simulink model "minseg_M2V3_2017a"  (R2017a)
settings: Solver=FixedStepDiscrete  StartTime=0.0  StopTime=inf  FixedStep=mdl_T_sample  RelTol=1e-3
undefined symbols (not defined in the file or in its folder): ctrl_lqr_K2, ctrl_motorDriver_v_ff_cmd_v_val, ctrl_motorDriver_v_ff_cmd_v_val_norm_dx_max, ctrl_motorDriver_v_ff_cmd_v_val_norm_dx_min, ctrl_motorDriver_v_output_max, ctrl_motorDriver_v_output_min, ctrl_motorDriver_v_pid_cmd_thetaDot_val, ctrl_motorDriver_v_pid_cmd_thetaDot_val_norm_dx_max, ctrl_motorDriver_v_pid_cmd_thetaDot_val_norm_dx_min, ctrl_motorDriver_v_pid_int_maxVal, ctrl_motorDriver_v_pid_int_minVal, ctrl_motorDriver_v_pid_k_d, ctrl_motorDriver_v_pid_k_i, ctrl_motorDriver_v_pid_k_p, ctrl_motorDriver_v_rts_ss_k_A, ctrl_motorDriver_v_rts_ss_k_B, ctrl_motorDriver_v_rts_ss_k_C, ctrl_motorDriver_v_rts_ss_k_D, ctrl_motorDriver_v_rts_ss_stateIC, ctrl_motorDriver_v_sfr_cmd_p_x_f, ctrl_motorDriver_v_sfr_cmd_p_x_mag, ctrl_motorDriver_v_sfr_cmd_p_y_f, ctrl_motorDriver_v_sfr_cmd_p_y_mag, ctrl_motorDriver_v_sfr_K, ctrl_motorDriver_v_sfr_K_plant, ctrl_motorDriver_v_sfr_K_rts, ctrl_motorDriver_v_T_cmd, ctrl_motorDriver_v_T_init, DiscIntNeverNeededParam, gyro_bias, io_srl_read_rateTransition_initialCondition, k_intmax_uint8, mdl_T_sample, mtr_encoder_filter_z_ss_A, mtr_encoder_filter_z_ss_B, mtr_encoder_filter_z_ss_C, mtr_encoder_filter_z_ss_D, plant, plant_accel_k_digital2analog, plant_body_l_c, plant_body_l_w, plant_gyro_encoder_filter_z_den, plant_gyro_encoder_filter_z_num, plant_gyro_filter_z_den, plant_gyro_filter_z_num, plant_gyro_k_digital2analog, plant_linear_ss_stateIC, plant_linear_ss_t_A, plant_linear_ss_t_B, plant_linear_ss_t_C, plant_linear_ss_t_D, plant_mtr_encoder_count2wheelRad, plant_mtr_encoder_filter_z_den, plant_mtr_encoder_filter_z_num, plant_pSupply_v, plant_supply_v, plant_T_init, plant_wheel_r
undefined symbols (not defined in the file): ctrl_lqr_addlDyn_A_discrete, ctrl_lqr_addlDyn_B_discrete, ctrl_lqr_addlDyn_C_discrete, ctrl_lqr_addlDyn_D_discrete, ctrl_lqr_addlDyn_k_antiWindup, ctrl_lqr_addlDyn_stateIC, plant_gyro_bias_movingAverage_n_pts, plant_linear_A_continuous, plant_linear_B_continuous, plant_linear_C_continuous, plant_linear_D_continuous, plant_linear_stateIC
libraries: svdutilitieslib x135, simulink x57, arduinolib x15, MinSegLibrary_M2V3 x3, dspindex x3, RASPlib x2
(part 1 of 6)
settings Model: ExtModeTrigDuration=2  Creator=kando  LastModifiedBy=kando
settings DataIOCC: SaveOutput=off  SignalLogging=off  DSMLogging=off  VisualizeSimOutput=off  SaveTime=off
settings OptimizationCC: LifeSpan=Inf  MaxStackSize=64  SimCompilerOptimization=on  AccelVerboseBuild=on
settings DebuggingCC: AllowSymbolicDim=off  SFUnexpectedBacktrackingDiag=warning  SFNoUnconditionalDefaultTransitionDiag=warning  SFExecutionAtInitializationDiag=none
settings HardwareCC: ProdBitPerInt=16  ProdBitPerPointer=16  ProdBitPerSizeT=16  ProdBitPerPtrDiffT=16  ProdLargestAtomicFloat=None  ProdWordSize=8  ProdHWDeviceType=Atmel->AVR  UseEmbeddedCoderFeatures=off  UseSimulinkCoderFeatures=off
settings ModelReferenceCC: PropagateSignalLabelsOutOfModel=off
settings SFSimCC: MATLABDynamicMemAlloc=off
settings RTWCC: SystemTargetFile=ert.tlc  HardwareBoard=Arduino Mega 2560  TLCOptions=-aInlineSetEventsForThisBaseRateFcn=TLC_FALSE -aSuppressMultiTaskScheduler=TLC_FALSE -aRateBasedStepFcn=1  TemplateMakefile=ert_default_tmf  Description=Embedded Coder  Toolchain=Arduino AVR  BuildConfiguration=Faster Runs
settings ERTTargetCC: MultiwordLength=2048  ERTCustomFileBanners=off  SupportContinuousTime=on  SupportNonInlinedSFcns=on  RemoveResetFunc=off  SupportVariableSizeSignals=on  ModelStepFunctionPrototypeControlCompliant=off  ConvertIfToSwitch=off  SuppressUnreachableDefaultCases=off
settings ConfigComp: CovMetricSettings=dw  CovHtmlReporting=on  CovSaveCumulativeToWorkspaceVar=on  CovSaveSingleToWorkspaceVar=on  CovExternalEMLEnable=off

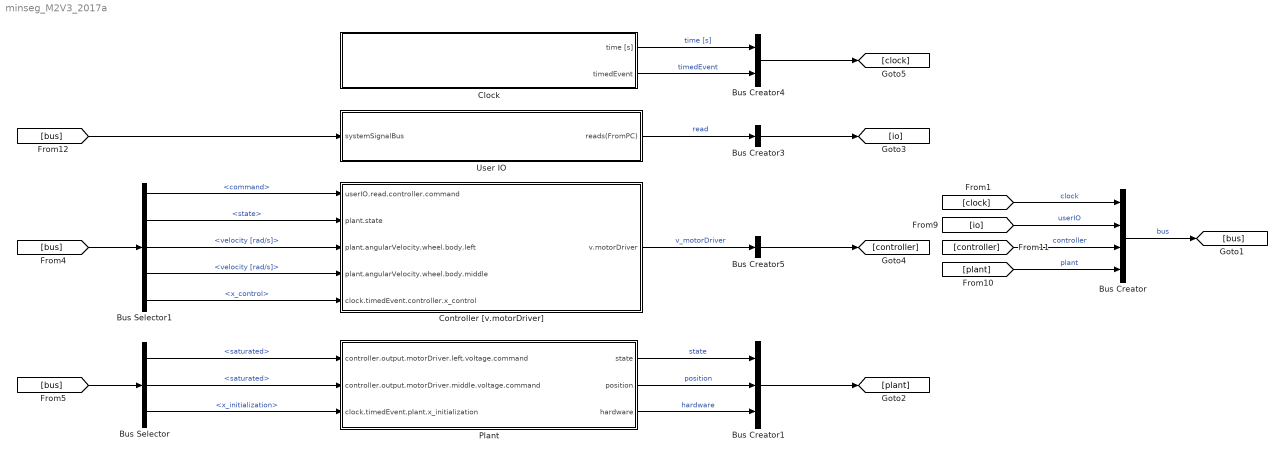
== system minseg_M2V3_2017a ==
  Bus Creator : BusCreator  Inputs=4
  Bus Creator1 : BusCreator  Inputs=3
  Bus Creator3 : BusCreator  Inputs=1
  Bus Creator4 : BusCreator  Inputs=2
  Bus Creator5 : BusCreator  Inputs=1
  Bus Selector : BusSelector  OutputSignals=controller.v_motorDriver.output.left.command [V].saturated,controller.v_motorDriver.output.middle.command [V].saturated,clock.timedEvent.plant.x_initialization
  Bus Selector1 : BusSelector  OutputSignals=userIO.read.controller.command,plant.state,plant.position.theta.body.left.velocity [rad/s],plant.position.theta.body.middle.velocity [rad/s],clock.timedEvent.controller.x_control
  Clock : Subsystem
  Controller [v.motorDriver] : Subsystem
  Plant : Subsystem  Variant=on  VariantControl=Variant1
  User IO : Subsystem
  wires:
  [io] -> Bus Creator/2  "userIO"
  [controller] -> Bus Creator/3  "controller"
  [plant] -> Bus Creator/4  "plant"
  Bus Creator/1 -> [bus]  "bus"
  Controller [v.motorDriver]/1(v.motorDriver) -> Bus Creator5/1  "v_motorDriver"
  [bus] -> User IO/1(systemSignalBus)
  Bus Creator3/1 -> [io]
  User IO/1(reads(FromPC)) -> Bus Creator3/1  "read"
  [bus] -> Bus Selector1/1
  [bus] -> Bus Selector/1
  Bus Creator1/1 -> [plant]
  Bus Creator4/1 -> [clock]
  [clock] -> Bus Creator/1  "clock"
  Plant/3(" hardware") -> Bus Creator1/3  "hardware"
  Clock/1(time [s]) -> Bus Creator4/1  "time [s]"
  Clock/2(timedEvent) -> Bus Creator4/2  "timedEvent"
  Bus Selector/1 -> Plant/1("controller.output.motorDriver.left.voltage.command ")  "<saturated>"
  Bus Selector/2 -> Plant/2("controller.output.motorDriver.middle.voltage.command ")  "<saturated>"
  Bus Selector/3 -> Plant/3(clock.timedEvent.plant.x_initialization)  "<x_initialization>"
  Plant/1(" state") -> Bus Creator1/1  "state"
  Plant/2(" position") -> Bus Creator1/2  "position"
  Bus Creator5/1 -> [controller]
  Bus Selector1/1 -> Controller [v.motorDriver]/1(userIO.read.controller.command)  "<command>"
  Bus Selector1/2 -> Controller [v.motorDriver]/2(plant.state)  "<state>"
  Bus Selector1/3 -> Controller [v.motorDriver]/3(plant.angularVelocity.wheel.body.left)  "<velocity [rad/s]>"
  Bus Selector1/4 -> Controller [v.motorDriver]/4(plant.angularVelocity.wheel.body.middle)  "<velocity [rad/s]>"
  Bus Selector1/5 -> Controller [v.motorDriver]/5(clock.timedEvent.controller.x_control)  "<x_control>"

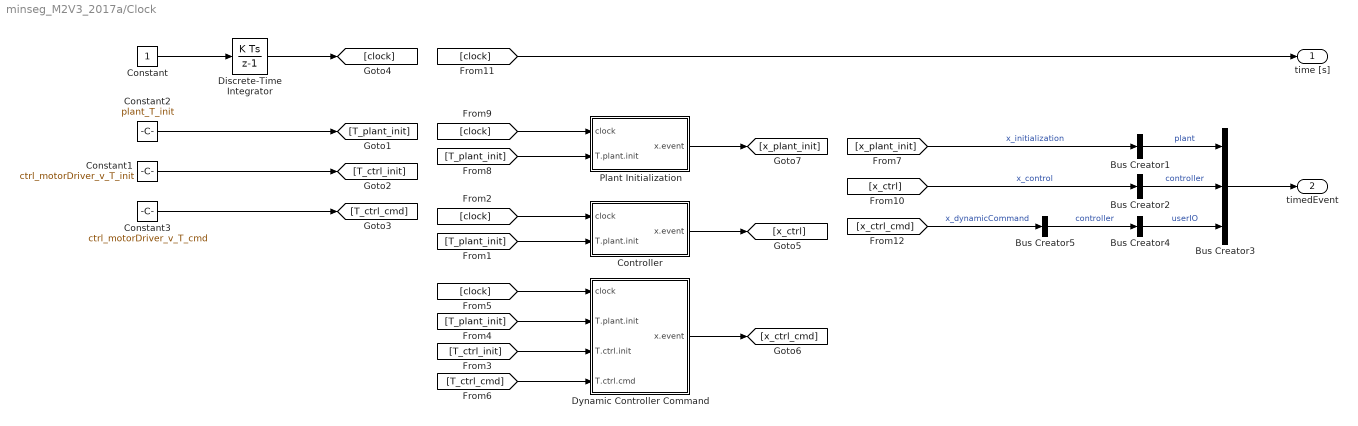
== system minseg_M2V3_2017a/Clock ==
  Bus Creator{1..2,4..5} (4 alike) : BusCreator  Inputs=1
  Bus Creator3 : BusCreator  Inputs=3
  Constant : Constant  SampleTime=mdl_T_sample
  Constant1 : Constant  Value=ctrl_motorDriver_v_T_init  SampleTime=mdl_T_sample
      settings: AttributesFormatString=%<Value>
  Constant2 : Constant  Value=plant_T_init  SampleTime=mdl_T_sample
      settings: AttributesFormatString=%<Value>
  Constant3 : Constant  Value=ctrl_motorDriver_v_T_cmd  SampleTime=mdl_T_sample
      settings: AttributesFormatString=%<Value>
  Controller : Subsystem
  Discrete-Time Integrator : DiscreteIntegrator  InitialConditionSetting=State (most efficient)  SampleTime=-1  ICPrevOutput=DiscIntNeverNeededParam  ICPrevScaledInput=DiscIntNeverNeededParam
  Dynamic Controller Command : Subsystem
  Plant Initialization : Subsystem
  time [s] : Outport
  timedEvent : Outport  Port=2
  wires:
  Bus Creator3/1 -> timedEvent/1
  Bus Creator1/1 -> Bus Creator3/1  "plant"
  [clock] -> time [s]/1
  Constant2/1 -> [T_plant_init]
  Constant1/1 -> [T_ctrl_init]
  [clock] -> Controller/1(clock)
  [T_plant_init] -> Controller/2(T.plant.init)
  [x_plant_init] -> Bus Creator1/1  "x_initialization"
  [x_ctrl] -> Bus Creator2/1  "x_control"
  [clock] -> Dynamic Controller Command/1(clock)
  [T_plant_init] -> Dynamic Controller Command/2(T.plant.init)
  [T_ctrl_init] -> Dynamic Controller Command/3(T.ctrl.init)
  Constant3/1 -> [T_ctrl_cmd]
  [T_ctrl_cmd] -> Dynamic Controller Command/4(T.ctrl.cmd)
  Controller/1(x.event) -> [x_ctrl]
  Dynamic Controller Command/1(x.event) -> [x_ctrl_cmd]
  Plant Initialization/1(x.event) -> [x_plant_init]
  [T_plant_init] -> Plant Initialization/2(T.plant.init)
  [clock] -> Plant Initialization/1(clock)
  [x_ctrl_cmd] -> Bus Creator5/1  "x_dynamicCommand"
  Bus Creator4/1 -> Bus Creator3/3  "userIO"
  Bus Creator5/1 -> Bus Creator4/1  "controller"
  Bus Creator2/1 -> Bus Creator3/2  "controller"
  Constant/1 -> Discrete-Time Integrator/1
  Discrete-Time Integrator/1 -> [clock]

== system minseg_M2V3_2017a/Controller [v.motorDriver] ==
  userIO.read.controller.command : Inport
  plant.state : Inport  Port=2
  plant.angularVelocity.wheel.body.left : Inport  Port=3
  plant.angularVelocity.wheel.body.middle : Inport  Port=4
  clock.timedEvent.controller.x_control : Inport  Port=5
  Archive : Subsystem  Commented=on
  Bus Creator2 : BusCreator  Inputs=2
  Controller and Enable : Subsystem
  Saturation : Subsystem
  v.motorDriver : Outport
  wires:
  Controller and Enable/2(error) -> Bus Creator2/2  "error"
  clock.timedEvent.controller.x_control/1 -> Controller and Enable/Enable
  userIO.read.controller.command/1 -> Controller and Enable/1(userIO.read.controller.command)
  plant.state/1 -> Controller and Enable/2(plant.state)
  plant.angularVelocity.wheel.body.left/1 -> Controller and Enable/3(plant.angularVelocity.wheel.body.left)
  plant.angularVelocity.wheel.body.middle/1 -> Controller and Enable/4(plant.angularVelocity.wheel.body.middle)
  Controller and Enable/1(output) -> Saturation/1(u.raw)
  Saturation/1(u.sat) -> Bus Creator2/1  "output"
  Bus Creator2/1 -> v.motorDriver/1

== system minseg_M2V3_2017a/Plant ==
  "controller.output.motorDriver.left.voltage.command " : Inport
  "controller.output.motorDriver.middle.voltage.command " : Inport  Port=2
  clock.timedEvent.plant.x_initialization : Inport  Port=3
  Hardware : Subsystem  VariantControl=(default)
  Hardware-Equivalent Linear Dynamics : Subsystem  VariantControl=plant_linearDynamics_var
  Hardware-Equivalent Nonlinear Dynamics : Subsystem  VariantControl=plant_nonlinearDynamics_var
  " state" : Outport
  " position" : Outport  Port=2
  " hardware" : Outport  Port=3

== system minseg_M2V3_2017a/User IO ==
  systemSignalBus : Inport
  Bus Creator1 : BusCreator  Inputs=1
  Bus Selector1 : BusSelector  OutputSignals=clock.timedEvent.userIO.controller.x_dynamicCommand
  Reads (From PC) : Subsystem
  Writes (To PC) : Subsystem  Variant=on  VariantControl=Variant1
  reads(FromPC) : Outport
  wires:
  Reads (From PC)/1(controller) -> Bus Creator1/1  "controller"
  systemSignalBus/1 -> Bus Selector1/1, Writes (To PC)/1("systemSignalBus ")
  Bus Creator1/1 -> reads(FromPC)/1
  Bus Selector1/1 -> Reads (From PC)/Enable  "<x_dynamicCommand>"

== system minseg_M2V3_2017a/Clock/Controller ==
  clock : Inport
  T.plant.init : Inport  Port=2
  Relational Operator1 : RelationalOperator  OutDataTypeStr=boolean  RndMeth=Simplest
  x.event : Outport
  wires:
  Relational Operator1/1 -> x.event/1
  clock/1 -> Relational Operator1/1
  T.plant.init/1 -> Relational Operator1/2

== system minseg_M2V3_2017a/Clock/Dynamic Controller Command ==
  clock : Inport
  T.plant.init : Inport  Port=2
  T.ctrl.init : Inport  Port=3
  T.ctrl.cmd : Inport  Port=4
  Add : Sum  Inputs=+++
  Add1 : Sum
  Logical Operator : Logic  AllPortsSameDT=off  OutDataTypeStr=boolean
  Relational Operator1 : RelationalOperator  OutDataTypeStr=boolean  RndMeth=Simplest
  Relational Operator2 : RelationalOperator  Operator=<  OutDataTypeStr=boolean  RndMeth=Simplest
  x.event : Outport
  wires:
  T.plant.init/1 -> [T_plant_init]
  T.ctrl.cmd/1 -> [T_ctrl_cmd]
  [T_plant_init] -> Add1/1
  [T_plant_init] -> Add/1
  [T_ctrl_cmd] -> Add/3
  Add/1 -> Relational Operator2/2
  clock/1 -> [clock]
  [clock] -> Relational Operator1/1
  [clock] -> Relational Operator2/1
  [T_ctrl_init] -> Add1/2
  T.ctrl.init/1 -> [T_ctrl_init]
  Add1/1 -> Relational Operator1/2
  [T_ctrl_init] -> Add/2
  Relational Operator2/1 -> Logical Operator/2
  Relational Operator1/1 -> Logical Operator/1
  Logical Operator/1 -> x.event/1

== system minseg_M2V3_2017a/Clock/Plant Initialization ==
  clock : Inport
  T.plant.init : Inport  Port=2
  Relational Operator1 : RelationalOperator  Operator=<  OutDataTypeStr=boolean  RndMeth=Simplest
  x.event : Outport
  wires:
  T.plant.init/1 -> Relational Operator1/2
  clock/1 -> Relational Operator1/1
  Relational Operator1/1 -> x.event/1

== system minseg_M2V3_2017a/Controller [v.motorDriver]/Archive ==
  Additional Dynamics: Reference Tracking : Subsystem  Commented=on  mask{A=ctrl_lqr_addlDyn_A_discrete, B=ctrl_lqr_addlDyn_B_discrete, C=ctrl_lqr_addlDyn_C_discrete, D=ctrl_lqr_addlDyn_D_discrete, state_initialCondition=ctrl_lqr_addlDyn_stateIC, k_antiWindup=ctrl_lqr_addlDyn_k_antiWindup}
      mask prompts: A "A Matrix"; B "B Matrix"; C "C Matrix"; D "D Matrix"; state_initialCondition "State Initial Condition"; k_antiWindup "Anti-windup Gain"
  Continuous State-Space : Subsystem  Commented=on  mask{A=ctrl_lqr_addlDyn_A_discrete, B=ctrl_lqr_addlDyn_B_discrete, C=ctrl_lqr_addlDyn_C_discrete, D=ctrl_lqr_addlDyn_D_discrete, state_initialCondition=ctrl_lqr_addlDyn_stateIC, k_antiWindup=ctrl_lqr_addlDyn_k_antiWindup}
      mask prompts: A "A Matrix"; B "B Matrix"; C "C Matrix"; D "D Matrix"; state_initialCondition "State Initial Condition"; k_antiWindup "Anti-windup Gain"
  From13 : From  Commented=on  GotoTag=x_sat
  From14 : From  Commented=on  GotoTag=KpXp
  From16 : From  Commented=on  GotoTag=output
  Goto9 : Goto  Commented=on  GotoTag=x_sat
  Limit Calculation : Subsystem  Commented=on
  Saturation : Saturate  Commented=on  UpperLimit=+1  LowerLimit=-1
  Saturation flag : Subsystem  Commented=on
  Terminator : Terminator  Commented=on
  wires:
  Limit Calculation/1(max(K.a•C.a•x.a)) -> ?
  From16/1 -> Saturation flag/1(u[k+1])
  Limit Calculation/2(min(K.a•C.a•x.a)) -> ?
  ? -> Goto9/1
  ? -> Terminator/1
  From14/1 -> Limit Calculation/1(K.plant•x.plant)

== system minseg_M2V3_2017a/Controller [v.motorDriver]/Controller and Enable ==
  userIO.read.controller.command : Inport
  plant.state : Inport  Port=2
  plant.angularVelocity.wheel.body.left : Inport  Port=3
  plant.angularVelocity.wheel.body.middle : Inport  Port=4
  Enable : EnablePort  StatesWhenEnabling=reset
  Controller : Subsystem  Variant=on  VariantControl=Variant1
  output : Outport
  error : Outport  Port=2
  wires:
  plant.state/1 -> Controller/2(plant.state)
  plant.angularVelocity.wheel.body.middle/1 -> Controller/4(plant.angularVelocity.wheel.body.middle)
  plant.angularVelocity.wheel.body.left/1 -> Controller/3(plant.angularVelocity.wheel.body.left)
  userIO.read.controller.command/1 -> Controller/1(userIO.read.controller.command)
  Controller/2(error) -> error/1
  Controller/1(output) -> output/1

== system minseg_M2V3_2017a/Controller [v.motorDriver]/Saturation ==
  u.raw : Inport
  Bus Creator{,1..3,5} (5 alike) : BusCreator  Inputs=2
  Constant1 : Constant  Value=ctrl_motorDriver_v_output_max  SampleTime=mdl_T_sample
      settings: AttributesFormatString=%<Value>
  Constant2 : Constant  Value=ctrl_motorDriver_v_output_min  SampleTime=mdl_T_sample
      settings: AttributesFormatString=%<Value>
  Demux : Demux  Outputs=2
  Left-Connected Motor : Subsystem
  Middle-Connected Motor : Subsystem
  u.sat : Outport
  wires:
  u.raw/1 -> Demux/1
  [u1] -> Left-Connected Motor/2(u.raw)
  Bus Creator2/1 -> Bus Creator5/1  "command [V]"
  [u_max] -> Left-Connected Motor/1(u.max)
  [u_min] -> Left-Connected Motor/3(u.min)
  Demux/1 -> [u1]
  Demux/2 -> [u2]
  Left-Connected Motor/2(x.saturating) -> Bus Creator5/2  "x_saturating"
  [u_min] -> Middle-Connected Motor/3(u.min)
  [u_max] -> Middle-Connected Motor/1(u.max)
  [u2] -> Middle-Connected Motor/2(u.raw)
  Bus Creator3/1 -> Bus Creator/2  "middle"
  Bus Creator5/1 -> Bus Creator/1  "left"
  Bus Creator/1 -> u.sat/1
  Constant1/1 -> [u_max]
  Constant2/1 -> [u_min]
  Left-Connected Motor/1(u.sat) -> Bus Creator2/2  "saturated"
  [u1] -> Bus Creator2/1  "raw"
  [u2] -> Bus Creator1/1  "raw"
  Middle-Connected Motor/1(u.sat) -> Bus Creator1/2  "saturated"
  Middle-Connected Motor/2(x.saturating) -> Bus Creator3/2  "x_saturating"
  Bus Creator1/1 -> Bus Creator3/1  "command [V]"

== system minseg_M2V3_2017a/Plant/Hardware ==
  "controller.output.motorDriver.left.voltage.command " : Inport
  "controller.output.motorDriver.middle.voltage.command " : Inport  Port=2
  clock.timedEvent.plant.x_initialization : Inport  Port=3
  Analog to Digital Conversion : Subsystem
  Arduino Pin IO : Subsystem
  Bus Creator1 : BusCreator  Inputs=3
  Bus Creator2 : BusCreator  Inputs=1
  Bus Creator3 : BusCreator  Inputs=2
  Bus Creator5 : BusCreator  Inputs=6
  Bus Creator6 : BusCreator  Inputs=2
  Bus Creator7 : BusCreator  Inputs=1
  Bus Creator8 : BusCreator  Inputs=1
  Bus Selector6 : BusSelector  OutputSignals=motorEncoder,gyroscope,accelerometer  OutputAsBus=on
  Calculations : Subsystem
  Digital to Analog Conversion : Subsystem
  State : Subsystem
  state : Outport
  position : Outport  Port=2
  hardware : Outport  Port=3
  wires:
  Bus Creator3/1 -> Bus Creator6/1  "digital"
  Analog to Digital Conversion/1(motorDriver) -> Bus Creator2/1  "motorDriver"
  Bus Creator2/1 -> [digitalPin_out]
  Arduino Pin IO/1(input(FromPins)) -> [digitalPin_in]
  "controller.output.motorDriver.left.voltage.command "/1 -> Analog to Digital Conversion/1(motorDriver.left.voltage.command)
  "controller.output.motorDriver.middle.voltage.command "/1 -> Analog to Digital Conversion/2(motorDriver.middle.voltage.command)
  [digitalPin_out] -> Arduino Pin IO/1(output(ToPins))
  [digitalPin_in] -> Bus Creator3/2  "in(FromPin)"
  [digitalPin_out] -> Bus Creator3/1  "out(ToPin)"
  [digitalPin_in] -> Digital to Analog Conversion/1(digitalInput)
  Digital to Analog Conversion/1(gyroscope) -> Bus Creator5/1  "gyroscope"
  Digital to Analog Conversion/2(accelerometer) -> Bus Creator5/2  "accelerometer"
  Digital to Analog Conversion/3(motorEncoder) -> Bus Creator5/3  "motorEncoder"
  Digital to Analog Conversion/4(pushbutton) -> Bus Creator5/4  "pushbutton"
  Digital to Analog Conversion/5(tempometer) -> Bus Creator5/5  "tempometer"
  Digital to Analog Conversion/6(magnetometer) -> Bus Creator5/6  "magnetometer"
  Bus Creator6/1 -> Bus Creator7/1  "pin"
  [analogPin_in] -> Bus Creator8/1  "in(FromPin)"
  Bus Creator5/1 -> [analogPin_in]
  Bus Creator7/1 -> hardware/1
  Bus Creator8/1 -> Bus Creator6/2  "analog"
  [analogPin_in] -> Bus Selector6/1
  Calculations/1(theta) -> Bus Creator1/1  "theta"
  Calculations/2(phi) -> Bus Creator1/2  "phi"
  Calculations/3(p) -> Bus Creator1/3  "p"
  Bus Creator1/1 -> State/1(data), position/1
  Bus Selector6/1 -> Calculations/1(analogInput)
  [x_model_init] -> Digital to Analog Conversion/2(clock.timedEvent.plant.x_initialization)
  clock.timedEvent.plant.x_initialization/1 -> [x_model_init]
  [x_model_init] -> Calculations/2(clock.timedEvent.plant.x_initialization)
  State/1(state) -> state/1

== system minseg_M2V3_2017a/Plant/Hardware-Equivalent Linear Dynamics ==
  "controller.output.motorDriver.left.voltage.command " : Inport
  "controller.output.motorDriver.middle.voltage.command " : Inport  Port=2
  Bus Creator1 : BusCreator  Inputs=3
  Bus Creator2 : BusCreator  Inputs=6
  Calculation : Subsystem
  Demux : Demux  Outputs=6
  Mux : Mux  Inputs=2
  Plant : StateSpace  A=plant_linear_ss_t_A  B=plant_linear_ss_t_B  C=plant_linear_ss_t_C  D=plant_linear_ss_t_D  X0=plant_linear_ss_stateIC
  Saturation : Saturate  UpperLimit=+plant_pSupply_v  LowerLimit=-plant_pSupply_v
      settings: AttributesFormatString=|
      | max: %<UpperLimit>
      | min: %<LowerLimit>
  Saturation1 : Saturate  UpperLimit=+plant_pSupply_v  LowerLimit=-plant_pSupply_v
      settings: AttributesFormatString=|
      | max: %<UpperLimit>
      | min: %<LowerLimit>
  State-Space : Subsystem  Commented=on  mask{A=plant_linear_A_continuous, B=plant_linear_B_continuous, C=plant_linear_C_continuous, D=plant_linear_D_continuous, integrator_initialCondition=plant_linear_stateIC}
      mask prompts: A "A Matrix"; B "B Matrix"; C "C Matrix"; D "D Matrix"; integrator_initialCondition "Integrator Initial Condition"
  Zero-Order Hold : ZeroOrderHold  SampleTime=mdl_T_sample
  state : Outport
  position : Outport  Port=2
  wires:
  "controller.output.motorDriver.left.voltage.command "/1 -> Saturation/1
  "controller.output.motorDriver.middle.voltage.command "/1 -> Saturation1/1
  Demux/1 -> Bus Creator2/1  "wheel_angularPosition_theta_global_average [rad]"
  Demux/4 -> Bus Creator2/4  "body_angularVelocity_phiDot_x [rad/s]"
  Demux/3 -> Bus Creator2/3  "wheel_angularVelocity_thetaDot_global_average [rad/s]"
  Demux/6 -> Bus Creator2/6  "body_angularVelocity_phiDot_y [rad/s]"
  Demux/2 -> Bus Creator2/2  "body_angularPosition_phi_x [rad]"
  Demux/5 -> Bus Creator2/5  "body_angularPosition_phi_y [rad]"
  Calculation/1(theta) -> Bus Creator1/1  "theta"
  Calculation/2(phi) -> Bus Creator1/2  "phi"
  Calculation/3(p) -> Bus Creator1/3  "p"
  Bus Creator1/1 -> position/1
  Zero-Order Hold/1 -> Demux/1
  Plant/1 -> Zero-Order Hold/1
  Mux/1 -> Plant/1
  Saturation/1 -> Mux/1
  Saturation1/1 -> Mux/2
  Bus Creator2/1 -> Calculation/1(plant.state), state/1

== system minseg_M2V3_2017a/Plant/Hardware-Equivalent Nonlinear Dynamics ==
  "controller.output.motorDriver.left.voltage.command " : Inport
  "controller.output.motorDriver.middle.voltage.command " : Inport  Port=2
  position : Outport
  wires:
  "controller.output.motorDriver.middle.voltage.command "/1 -> ?
  "controller.output.motorDriver.left.voltage.command "/1 -> ?

== system minseg_M2V3_2017a/User IO/Reads (From PC) ==
  Enable : EnablePort
  Bus Creator1 : BusCreator  Inputs=1
  Constant : Constant  SampleTime=mdl_T_sample
  Controller : Subsystem  Variant=on  VariantControl=Variant1
  Discrete-Time Integrator : DiscreteIntegrator  InitialConditionSetting=State (most efficient)  SampleTime=-1  ICPrevOutput=DiscIntNeverNeededParam  ICPrevScaledInput=DiscIntNeverNeededParam
  controller : Outport
  wires:
  Controller/1(command) -> Bus Creator1/1  "command"
  Bus Creator1/1 -> controller/1
  Discrete-Time Integrator/1 -> Controller/1(clock.userIO)
  Constant/1 -> Discrete-Time Integrator/1

== system minseg_M2V3_2017a/User IO/Writes (To PC) ==
  "systemSignalBus " : Inport
  Plant: Hardware : Subsystem  Variant=on  VariantControl=(default)
  Plant: Linear Dynamics : Subsystem  Variant=on  VariantControl=plant_linearDynamics_var
  Plant: Nonlinear Dynamics : Subsystem  Variant=on  VariantControl=plant_nonlinearDynamics_var

== system minseg_M2V3_2017a/Controller [v.motorDriver]/Archive/Additional Dynamics: Reference Tracking ==
  u : Inport
  max(K•C•x) : Inport  Port=2
  min(K•C•x) : Inport  Port=3
  reset : Inport  Port=4
  Add : Sum
  Add1 : Sum
  Delay : Subsystem
  Gain : Gain  Gain=A  Multiplication=Matrix(K*u)
  Gain1 : Gain  Gain=B  Multiplication=Matrix(K*u)
  Gain2 : Gain  Gain=C  Multiplication=Matrix(K*u)
  Gain3 : Gain  Commented=on  Gain=D  Multiplication=Matrix(K*u)
  y : Outport
  x : Outport  Port=2
  x.sat : Outport  Port=3
  wires:
  Gain1/1 -> Add/2
  Gain3/1 -> Add1/2
  Gain2/1 -> Add1/1
  Gain/1 -> Add/1
  u/1 -> Gain3/1, Gain1/1  "u[k]"
  Add1/1 -> y/1  "y"
  Delay/1(x[k]) -> Gain2/1, x/1, Gain/1  "x[k]"
  Add/1 -> Delay/1(x[k+1])  "x[k+1]"
  Delay/2(x.sat) -> x.sat/1
  max(K•C•x)/1 -> Delay/2(max(K•C•x))
  min(K•C•x)/1 -> Delay/3(min(K•C•x))
  reset/1 -> Delay/4(reset)

== system minseg_M2V3_2017a/Controller [v.motorDriver]/Archive/Continuous State-Space ==
  u : Inport
  max(K•C•x) : Inport  Port=2
  min(K•C•x) : Inport  Port=3
  reset : Inport  Port=4
  Add : Sum
  Add1 : Sum
  Gain : Gain  Gain=A  Multiplication=Matrix(K*u)
  Gain1 : Gain  Gain=B  Multiplication=Matrix(K*u)
  Gain2 : Gain  Gain=C  Multiplication=Matrix(K*u)
  Gain3 : Gain  Commented=on  Gain=D  Multiplication=Matrix(K*u)
  Integrator : Subsystem
  y : Outport
  x : Outport  Port=2
  x.sat : Outport  Port=3
  wires:
  reset/1 -> Integrator/4(reset)
  min(K•C•x)/1 -> Integrator/3(min(K•C•x))
  max(K•C•x)/1 -> Integrator/2(max(K•C•x))
  Integrator/2(x.sat) -> x.sat/1
  Add/1 -> Integrator/1(x.dot)  "x.dot"
  Integrator/1(x) -> x/1, Gain/1, Gain2/1  "x"
  Add1/1 -> y/1  "y"
  u/1 -> Gain1/1, Gain3/1  "u"
  Gain/1 -> Add/1
  Gain2/1 -> Add1/1
  Gain3/1 -> Add1/2
  Gain1/1 -> Add/2

== system minseg_M2V3_2017a/Controller [v.motorDriver]/Archive/Limit Calculation ==
  note: -K.p•x.p + -K.a •y.a = y
      | -K.p•x.p + -K.a •C.a•x.a = y
      | -K.p•x.p + -K.a •I •x.a = y
      | -K.p•x.p + -K.a •x.a = y
      |
      | y ≥ -v.nom
      | -K.a•x.a + -K.p •x.p ≥ -v.nom
      | K.a•x.a + K.p •x.p ≤ v.nom
      | K.a•x.a ≤ -K.p •x.p + v.nom
      | K.a•x.a ≤ max(K.a•x.a)
      |
      | y ≤ v.nom
      | -K.a•x.a + -K.p •x.p ≤ v.nom
      | K.a•x.a + K.p •x.p ≥ -v.nom
      | K.a•x.a ≥ -K.p •x.p + -v.nom
      | K.a•x.a ≥ min(K.a•x.a)
  K.plant•x.plant : Inport
  Add2 : Sum  Inputs=--
  Add3 : Sum  Inputs=+-
  Constant1 : Constant  Value=plant_supply_v  SampleTime=mdl_T_sample
      settings: AttributesFormatString=%<Value>
  max(K.a•C.a•x.a) : Outport
  min(K.a•C.a•x.a) : Outport  Port=2
  wires:
  Add3/1 -> max(K.a•C.a•x.a)/1
  [v_nom] -> Add2/1
  [KpXp] -> Add2/2
  Add2/1 -> min(K.a•C.a•x.a)/1
  K.plant•x.plant/1 -> [KpXp]
  [KpXp] -> Add3/2
  Constant1/1 -> [v_nom]
  [v_nom] -> Add3/1

== system minseg_M2V3_2017a/Controller [v.motorDriver]/Archive/Saturation flag ==
  u[k+1] : Inport
  u.max : Inport  Port=2
  u.min : Inport  Port=3
  Add : Sum
  Data Type Conversion : DataTypeConversion  OutDataTypeStr=uint8
  Data Type Conversion1 : DataTypeConversion  OutDataTypeStr=uint8
  Gain : Gain  Gain=uint8(1)  OutDataTypeStr=uint8
      settings: AttributesFormatString=%<Gain>
  Gain1 : Gain  Gain=uint8(2)  OutDataTypeStr=uint8
      settings: AttributesFormatString=%<Gain>
  Relational Operator : RelationalOperator  OutDataTypeStr=boolean  RndMeth=Nearest
  Relational Operator1 : RelationalOperator  Operator=<=  OutDataTypeStr=boolean  RndMeth=Nearest
  x.saturating : Outport
  wires:
  u[k+1]/1 -> [u_kp1]
  [u_kp1] -> Relational Operator/1
  u.max/1 -> Relational Operator/2
  [u_kp1] -> Relational Operator1/1
  u.min/1 -> Relational Operator1/2
  Add/1 -> x.saturating/1  "x.saturating"
  Relational Operator1/1 -> Data Type Conversion1/1  "x.lowerSaturating"
  Relational Operator/1 -> Data Type Conversion/1  "x.upperSaturating"
  Data Type Conversion/1 -> Gain/1
  Data Type Conversion1/1 -> Gain1/1
  Gain/1 -> Add/1
  Gain1/1 -> Add/2

== system minseg_M2V3_2017a/Controller [v.motorDriver]/Controller and Enable/Controller ==
  userIO.read.controller.command : Inport
  plant.state : Inport  Port=2
  plant.angularVelocity.wheel.body.left : Inport  Port=3
  plant.angularVelocity.wheel.body.middle : Inport  Port=4
  Feed-Forward : Subsystem  VariantControl=ctrl_motorDriver_v_ff_var
  PID : Subsystem  VariantControl=ctrl_motorDriver_v_pid_var
  State Feedback Regulation : Subsystem  VariantControl=ctrl_motorDriver_v_sfr_var
  State Feedback Regulation with Reference Tracking System : Subsystem  VariantControl=(default)
  output : Outport
  error : Outport  Port=2

== system minseg_M2V3_2017a/Controller [v.motorDriver]/Saturation/Left-Connected Motor ==
  u.max : Inport
  u.raw : Inport  Port=2
  u.min : Inport  Port=3
  Saturation Dynamic : simulink/Discontinuities/Saturation Dynamic  OutMin=[]  OutMax=[]  OutDataTypeStr=Inherit: Same as second input  OutDataType=fixdt(1, 16)  OutScaling=2^-10  DoSatur=off
  Saturation flag : Subsystem
  u.sat : Outport
  x.saturating : Outport  Port=2
  wires:
  Saturation Dynamic/1 -> u.sat/1
  u.max/1 -> [u_max]
  u.raw/1 -> [u_raw]
  u.min/1 -> [u_min]
  [u_min] -> Saturation Dynamic/3
  [u_raw] -> Saturation Dynamic/2
  [u_max] -> Saturation Dynamic/1
  Saturation flag/1(x.saturating) -> x.saturating/1
  [u_max] -> Saturation flag/1(u.max)
  [u_raw] -> Saturation flag/2(u.raw)
  [u_min] -> Saturation flag/3(u.min)

== system minseg_M2V3_2017a/Controller [v.motorDriver]/Saturation/Middle-Connected Motor ==
  u.max : Inport
  u.raw : Inport  Port=2
  u.min : Inport  Port=3
  Saturation Dynamic : simulink/Discontinuities/Saturation Dynamic  OutMin=[]  OutMax=[]  OutDataTypeStr=Inherit: Same as second input  OutDataType=fixdt(1, 16)  OutScaling=2^-10  DoSatur=off
  Saturation flag : Subsystem
  u.sat : Outport
  x.saturating : Outport  Port=2
  wires:
  [u_min] -> Saturation flag/3(u.min)
  [u_raw] -> Saturation flag/2(u.raw)
  [u_max] -> Saturation flag/1(u.max)
  Saturation flag/1(x.saturating) -> x.saturating/1
  [u_max] -> Saturation Dynamic/1
  [u_raw] -> Saturation Dynamic/2
  [u_min] -> Saturation Dynamic/3
  u.min/1 -> [u_min]
  u.raw/1 -> [u_raw]
  u.max/1 -> [u_max]
  Saturation Dynamic/1 -> u.sat/1

== system minseg_M2V3_2017a/Plant/Hardware/Analog to Digital Conversion ==
  motorDriver.left.voltage.command : Inport
  motorDriver.middle.voltage.command : Inport  Port=2
  Bus Creator2 : BusCreator  Inputs=2
  Motor Driver : Subsystem
  motorDriver : Outport
  wires:
  motorDriver.middle.voltage.command/1 -> Motor Driver/2(middle.voltage.command)
  motorDriver.left.voltage.command/1 -> Motor Driver/1(left.voltage.command)
  Bus Creator2/1 -> motorDriver/1
  Motor Driver/1(left) -> Bus Creator2/1  "left"
  Motor Driver/2(middle) -> Bus Creator2/2  "middle"

== system minseg_M2V3_2017a/Plant/Hardware/Arduino Pin IO ==
  output(ToPins) : Inport
  Bus Creator6 : BusCreator  Inputs=6
  Bus Selector1 : BusSelector  OutputSignals=motorDriver.left.voltage.command.digital.positive [V],motorDriver.left.voltage.command.digital.negative [V],motorDriver.middle.voltage.command.digital.positive [V],motorDriver.middle.voltage.command.digital.negative [V]
  Digital Inputs (Reads from Pins) : Subsystem
  Digital Outputs (Writes to Pins) : Subsystem
  input(FromPins) : Outport
  wires:
  Digital Inputs (Reads from Pins)/1(gyroscope) -> Bus Creator6/1  "gyroscope"
  Digital Inputs (Reads from Pins)/2(accelerometer) -> Bus Creator6/2  "accelerometer"
  Digital Inputs (Reads from Pins)/3(motorEncoder) -> Bus Creator6/3  "motorEncoder"
  Digital Inputs (Reads from Pins)/4(magnetometer) -> Bus Creator6/4  "magnetometer"
  Digital Inputs (Reads from Pins)/5(pushbutton) -> Bus Creator6/5  "pushbutton"
  Digital Inputs (Reads from Pins)/6(tempometer) -> Bus Creator6/6  "tempometer"
  Bus Creator6/1 -> input(FromPins)/1
  output(ToPins)/1 -> Bus Selector1/1
  Bus Selector1/1 -> Digital Outputs (Writes to Pins)/1(motorDriver.left.voltage.command.digital.positive)  "<positive [V]>"
  Bus Selector1/2 -> Digital Outputs (Writes to Pins)/2(motorDriver.left.voltage.command.digital.negative)  "<negative [V]>"
  Bus Selector1/3 -> Digital Outputs (Writes to Pins)/3(motorDriver.middle.voltage.command.digital.positive)  "<positive [V]>"
  Bus Selector1/4 -> Digital Outputs (Writes to Pins)/4(motorDriver.middle.voltage.command.digital.negative)  "<negative [V]>"

== system minseg_M2V3_2017a/Plant/Hardware/Calculations ==
  analogInput : Inport
  clock.timedEvent.plant.x_initialization : Inport  Port=2
  Body Angular Position (phi) : Subsystem
  Bus Creator1 : BusCreator  Inputs=3
  Bus Creator4 : BusCreator  Inputs=2
  Bus Creator6 : BusCreator  Inputs=2
  Bus Selector1 : BusSelector  OutputSignals=motorEncoder.left [rad],motorEncoder.middle [rad]
  Bus Selector2 : BusSelector  OutputSignals=gyroscope.x [rad/s],gyroscope.y [rad/s],gyroscope.z [rad/s],accelerometer.x [rad/s^2],accelerometer.y [rad/s^2],accelerometer.z [rad/s^2]
  Bus Selector3 : BusSelector  OutputSignals=global.middle.velocity [rad/s]
  Bus Selector4 : BusSelector  OutputSignals=global.left.position [rad],global.middle.position [rad]
  Bus Selector5 : BusSelector  OutputSignals=x (pitch).position [rad],y (yaw).position [rad]
  Bus Selector6 : BusSelector  OutputSignals=x (pitch).position [rad]
  Linear Position (p) : Subsystem
  Wheel Angular Position (theta) : Subsystem
  theta : Outport
  phi : Outport  Port=2
  p : Outport  Port=3
  wires:
  Body Angular Position (phi)/3(z) -> Bus Creator1/3  "z (roll)"
  Bus Creator6/1 -> p/1
  Linear Position (p)/2(body) -> Bus Creator6/2  "body"
  Linear Position (p)/1(wheel) -> Bus Creator6/1  "wheel"
  Body Angular Position (phi)/1(x) -> Bus Creator1/1  "x (pitch)"
  Body Angular Position (phi)/2(y) -> Bus Creator1/2  "y (yaw)"
  Bus Creator1/1 -> [phi], phi/1
  Wheel Angular Position (theta)/2(global) -> Bus Creator4/2  "global"
  Wheel Angular Position (theta)/1(body) -> Bus Creator4/1  "body"
  analogInput/1 -> [analog]
  [analog] -> Bus Selector1/1
  [analog] -> Bus Selector2/1
  [theta] -> Bus Selector3/1
  Bus Selector1/1 -> Wheel Angular Position (theta)/1(motorEncoder.left)  "<left [rad]>"
  Bus Selector1/2 -> Wheel Angular Position (theta)/2(motorEncoder.middle)  "<middle [rad]>"
  Bus Selector2/2 -> Body Angular Position (phi)/2(gyroscope.y)  "<y [rad/s]>"
  Bus Selector2/1 -> Body Angular Position (phi)/1(gyroscope.x)  "<x [rad/s]>"
  Bus Selector2/3 -> Body Angular Position (phi)/3(gyroscope.z)  "<z [rad/s]>"
  Bus Selector2/4 -> Body Angular Position (phi)/4(accelerometer.x)  "<x [rad/s^2]>"
  Bus Selector2/5 -> Body Angular Position (phi)/5(accelerometer.y)  "<y [rad/s^2]>"
  Bus Selector2/6 -> Body Angular Position (phi)/6(accelerometer.z)  "<z [rad/s^2]>"
  [phi] -> Bus Selector6/1
  Bus Creator4/1 -> [theta], theta/1
  [theta] -> Bus Selector4/1
  [phi] -> Bus Selector5/1
  Bus Selector3/1 -> Linear Position (p)/1(wheel.angularVelocity.global)  "<velocity [rad/s]>"
  Bus Selector5/2 -> Linear Position (p)/3(body.angularPosition.y (yaw))  "<position [rad]>"
  Bus Selector5/1 -> Linear Position (p)/2(body.angularPosition.x (pitch))  "<position [rad]>"
  Bus Selector6/1 -> Wheel Angular Position (theta)/3(body.angularPosition.x (pitch))  "<position [rad]>"
  Bus Selector4/1 -> Body Angular Position (phi)/7(wheel.angularPosition.global.left)  "<position [rad]>"
  Bus Selector4/2 -> Body Angular Position (phi)/8(wheel.angularPosition.global.middle)  "<position [rad]>"
  clock.timedEvent.plant.x_initialization/1 -> [x_init]
  [x_init] -> Body Angular Position (phi)/9(clock.timedEvent.plant.x_initialization)

== system minseg_M2V3_2017a/Plant/Hardware/Digital to Analog Conversion ==
  digitalInput : Inport
  clock.timedEvent.plant.x_initialization : Inport  Port=2
  Accelerometer : Subsystem
  Bus Creator1 : BusCreator  Inputs=3
  Bus Creator2 : BusCreator  Inputs=3
  Bus Creator3 : BusCreator  Inputs=2
  Bus Creator4 : BusCreator  Inputs=3
  Bus Selector1 : BusSelector  OutputSignals=gyroscope.x.digital [-],gyroscope.y.digital [-],gyroscope.z.digital [-]
  Bus Selector3 : BusSelector  OutputSignals=gyroscope.x.digital [-],gyroscope.y.digital [-],gyroscope.z.digital [-]
  Bus Selector4 : BusSelector  OutputSignals=motorEncoder.left.digital [-],motorEncoder.middle.digital [-]
  Bus Selector5 : BusSelector  OutputSignals=gyroscope.x.digital [-],gyroscope.y.digital [-],gyroscope.z.digital [-]
  Bus Selector6 : BusSelector  OutputSignals=gyroscope.x.digital [-]
  Bus Selector7 : BusSelector  OutputSignals=gyroscope.x.digital [-]
  Gyroscope : Subsystem
  Magnetometer (Incomplete) : Subsystem
  Motor Encoder : Subsystem
  Pushbutton (Incomplete) : Subsystem
  Tempometer (Incomplete) : Subsystem
  gyroscope : Outport
  accelerometer : Outport  Port=2
  motorEncoder : Outport  Port=3
  pushbutton : Outport  Port=4
  tempometer : Outport  Port=5
  magnetometer : Outport  Port=6
  wires:
  Bus Creator2/1 -> gyroscope/1
  Bus Selector1/1 -> Gyroscope/1(x.digital)  "<digital [-]>"
  Bus Selector1/2 -> Gyroscope/2(y.digital)  "<digital [-]>"
  Bus Selector1/3 -> Gyroscope/3(z.digital)  "<digital [-]>"
  Gyroscope/1(x.analog) -> Bus Creator2/1  "x [rad/s]"
  Gyroscope/2(y.analog) -> Bus Creator2/2  "y [rad/s]"
  Gyroscope/3(z.analog) -> Bus Creator2/3  "z [rad/s]"
  digitalInput/1 -> [digital]
  [digital] -> Bus Selector1/1
  Accelerometer/3(z.analog) -> Bus Creator1/3  "z [rad/s^2]"
  Accelerometer/2(y.analog) -> Bus Creator1/2  "y [rad/s^2]"
  Accelerometer/1(x.analog) -> Bus Creator1/1  "x [rad/s^2]"
  Bus Creator1/1 -> accelerometer/1
  [digital] -> Bus Selector3/1
  Bus Selector3/3 -> Accelerometer/3(z.digital)  "<digital [-]>"
  Bus Selector3/2 -> Accelerometer/2(y.digital)  "<digital [-]>"
  Bus Selector3/1 -> Accelerometer/1(x.digital)  "<digital [-]>"
  Bus Selector4/1 -> Motor Encoder/1(left.digital)  "<digital [-]>"
  Bus Selector4/2 -> Motor Encoder/2(middle.digital)  "<digital [-]>"
  [digital] -> Bus Selector4/1
  [digital] -> Bus Selector5/1
  Bus Selector5/3 -> Magnetometer (Incomplete)/3(z.digital)  "<digital [-]>"
  Bus Selector5/2 -> Magnetometer (Incomplete)/2(y.digital)  "<digital [-]>"
  Bus Selector5/1 -> Magnetometer (Incomplete)/1(x.digital)  "<digital [-]>"
  [digital] -> Bus Selector6/1
  Bus Selector6/1 -> Pushbutton (Incomplete)/1(digital)  "<digital [-]>"
  Bus Selector7/1 -> Tempometer (Incomplete)/1(digital)  "<digital [-]>"
  [digital] -> Bus Selector7/1
  Motor Encoder/2(middle.analog) -> Bus Creator3/2  "middle [rad]"
  Motor Encoder/1(left.analog) -> Bus Creator3/1  "left [rad]"
  Bus Creator3/1 -> motorEncoder/1
  Bus Creator4/1 -> magnetometer/1
  Magnetometer (Incomplete)/1(x.analog) -> Bus Creator4/1  "x [?]"
  Magnetometer (Incomplete)/2(y.analog) -> Bus Creator4/2  "y [?]"
  Magnetometer (Incomplete)/3(z.analog) -> Bus Creator4/3  "z [?]"
  Pushbutton (Incomplete)/1(analog) -> pushbutton/1
  Tempometer (Incomplete)/1(analog) -> tempometer/1
  clock.timedEvent.plant.x_initialization/1 -> [x_init]
  [x_init] -> Gyroscope/4(clock.timedEvent.plant.x_initialization)

== system minseg_M2V3_2017a/Plant/Hardware/State ==
  data : Inport
  Bus Creator4 : BusCreator  Inputs=6
  Bus Selector1 : BusSelector  OutputSignals=theta.global.average.position [rad],phi.x (pitch).position [rad],theta.global.average.velocity [rad/s],phi.x (pitch).velocity [rad/s],phi.y (yaw).position [rad],phi.y (yaw).velocity [rad/s]
  state : Outport
  wires:
  data/1 -> Bus Selector1/1
  [theta] -> Bus Creator4/1  "wheel_angularPosition_theta_global_average [rad]"
  [phi_y] -> Bus Creator4/5  "body_angularPosition_phi_y [rad]"
  [theta_dot] -> Bus Creator4/3  "wheel_angularVelocity_thetaDot_global_average [rad/s]"
  Bus Creator4/1 -> state/1
  [phi_y_dot] -> Bus Creator4/6  "body_angularVelocity_phiDot_y [rad/s]"
  [phi_x] -> Bus Creator4/2  "body_angularPosition_phi_x [rad]"
  [phi_x_dot] -> Bus Creator4/4  "body_angularVelocity_phiDot_x [rad/s]"
  Bus Selector1/1 -> [theta]  "<position [rad]>"
  Bus Selector1/2 -> [phi_x]  "<position [rad]>"
  Bus Selector1/3 -> [theta_dot]  "<velocity [rad/s]>"
  Bus Selector1/4 -> [phi_x_dot]  "<velocity [rad/s]>"
  Bus Selector1/5 -> [phi_y]  "<position [rad]>"
  Bus Selector1/6 -> [phi_y_dot]  "<velocity [rad/s]>"

== system minseg_M2V3_2017a/Plant/Hardware-Equivalent Linear Dynamics/Calculation ==
  plant.state : Inport
  Bus Creator{1..4,6} (5 alike) : BusCreator  Inputs=2
  Bus Selector : BusSelector  OutputSignals=wheel_angularPosition_theta_global_average [rad],body_angularPosition_phi_x [rad],wheel_angularVelocity_thetaDot_global_average [rad/s],body_angularVelocity_phiDot_x [rad/s],body_angularPosition_phi_y [rad],body_angularVelocity_phiDot_y [rad/s]
  Linear Position (p) : Subsystem
  Wheel Angular Position (theta) : Subsystem
  theta : Outport
  phi : Outport  Port=2
  p : Outport  Port=3
  wires:
  [phi_y] -> Wheel Angular Position (theta)/4(body.angularPosition.y (yaw))
  Bus Selector/1 -> [theta]  "<wheel_angularPosition_theta_global_average [rad]>"
  Bus Selector/2 -> [phi_x]  "<body_angularPosition_phi_x [rad]>"
  Bus Selector/5 -> [phi_y]  "<body_angularPosition_phi_y [rad]>"
  Bus Selector/4 -> [phi_x_dot]  "<body_angularVelocity_phiDot_x [rad/s]>"
  [theta] -> Wheel Angular Position (theta)/1(wheel.angularPosition.global.average)
  [phi_x] -> Bus Creator3/1  "position [rad]"
  [phi_x_dot] -> Bus Creator3/2  "velocity [rad/s]"
  [phi_y_dot] -> Bus Creator4/2  "velocity [rad/s]"
  [phi_x] -> Linear Position (p)/2(body.angularPosition.x (pitch))
  [phi_x] -> Wheel Angular Position (theta)/3(body.angularPosition.x (pitch))
  [phi_y] -> Bus Creator4/1  "position [rad]"
  Bus Creator2/1 -> phi/1
  [theta_dot] -> Linear Position (p)/1(wheel.angularVelocity.global)
  [phi_y] -> Linear Position (p)/3(body.angularPosition.y (yaw))
  Wheel Angular Position (theta)/1(body) -> Bus Creator1/1  "body"
  Bus Selector/6 -> [phi_y_dot]  "<body_angularVelocity_phiDot_y [rad/s]>"
  Bus Selector/3 -> [theta_dot]  "<wheel_angularVelocity_thetaDot_global_average [rad/s]>"
  Wheel Angular Position (theta)/2(global) -> Bus Creator1/2  "global"
  Bus Creator4/1 -> Bus Creator2/2  "y (yaw)"
  Bus Creator3/1 -> Bus Creator2/1  "x (pitch)"
  Linear Position (p)/2(body) -> Bus Creator6/2  "body"
  Linear Position (p)/1(wheel) -> Bus Creator6/1  "wheel"
  Bus Creator6/1 -> p/1
  Bus Creator1/1 -> theta/1
  [theta_dot] -> Wheel Angular Position (theta)/2(wheel.angularVelocity.global.average)
  plant.state/1 -> Bus Selector/1

== system minseg_M2V3_2017a/Plant/Hardware-Equivalent Linear Dynamics/State-Space ==
  u : Inport
  Add : Sum
  Add1 : Sum
  Gain : Gain  Gain=A  Multiplication=Matrix(K*u)
  Gain1 : Gain  Gain=B  Multiplication=Matrix(K*u)
  Gain2 : Gain  Gain=C  Multiplication=Matrix(K*u)
  Gain3 : Gain  Commented=on  Gain=D  Multiplication=Matrix(K*u)
  Integrator : Integrator  InitialCondition=integrator_initialCondition
      settings: AttributesFormatString=initialCondition = %<InitialCondition>
  y : Outport
  x : Outport  Port=2
  wires:
  Gain1/1 -> Add/2
  Integrator/1 -> Gain2/1, x/1, Gain/1  "x"
  Gain3/1 -> Add1/2
  Gain2/1 -> Add1/1
  Gain/1 -> Add/1
  Add/1 -> Integrator/1  "x.dot"
  u/1 -> Gain3/1, Gain1/1  "u"
  Add1/1 -> y/1  "y"

== system minseg_M2V3_2017a/User IO/Reads (From PC)/Controller ==
  clock.userIO : Inport
  Feed-Forward : Subsystem  VariantControl=ctrl_motorDriver_v_ff_var
  PID : Subsystem  VariantControl=ctrl_motorDriver_v_pid_var
  State Feedback Regulation : Subsystem  VariantControl=(default)
  command : Outport

== system minseg_M2V3_2017a/User IO/Writes (To PC)/Plant: Hardware ==
  "systemSignalBus " : Inport
  Controller: FF : Subsystem  VariantControl=ctrl_motorDriver_v_ff_var
  Controller: PID : Subsystem  Variant=on  VariantControl=ctrl_motorDriver_v_pid_var
  Controller: SFR : Subsystem  Variant=on  VariantControl=(default)

== system minseg_M2V3_2017a/User IO/Writes (To PC)/Plant: Linear Dynamics ==
  "systemSignalBus " : Inport
  Controller: FF : Subsystem  Variant=on  VariantControl=ctrl_motorDriver_v_ff_var
  Controller: PID : Subsystem  Variant=on  VariantControl=ctrl_motorDriver_v_pid_var
  Controller: SFR : Subsystem  VariantControl=(default)

== system minseg_M2V3_2017a/User IO/Writes (To PC)/Plant: Nonlinear Dynamics ==
  "systemSignalBus " : Inport
  Controller: FF : Subsystem  Variant=on  VariantControl=ctrl_motor_v_ff_var  OverrideUsingVariant=(default)
  Controller: PID : Subsystem  Variant=on  VariantControl=(default)  OverrideUsingVariant=(default)

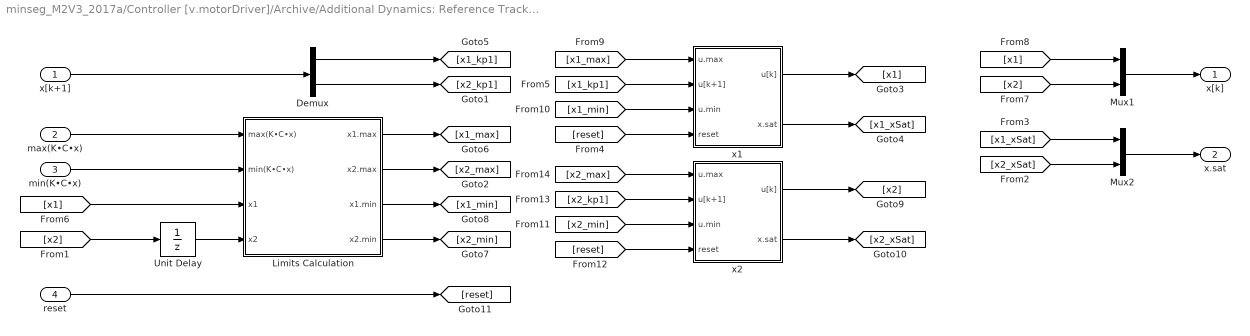
== system minseg_M2V3_2017a/Controller [v.motorDriver]/Archive/Additional Dynamics: Reference Tracking/Delay ==
  x[k+1] : Inport
  max(K•C•x) : Inport  Port=2
  min(K•C•x) : Inport  Port=3
  reset : Inport  Port=4
  Demux : Demux  Outputs=2
  Limits Calculation : Subsystem
  Mux1 : Mux  Inputs=2
  Mux2 : Mux  Inputs=2
  Unit Delay : UnitDelay  SampleTime=-1
  x1 : Subsystem  mask{u_init=state_initialCondition(1,1), k_antiWindup=k_antiWindup(1,1)}
      mask prompts: u_init "Initial Condition"; k_antiWindup "Anti-windup Gain"
  x2 : Subsystem  mask{u_init=state_initialCondition(2,1), k_antiWindup=k_antiWindup(2,1)}
      mask prompts: u_init "Initial Condition"; k_antiWindup "Anti-windup Gain"
  x[k] : Outport
  x.sat : Outport  Port=2
  wires:
  x[k+1]/1 -> Demux/1
  Demux/1 -> [x1_kp1]
  Demux/2 -> [x2_kp1]
  [x1] -> Mux1/1
  [x2] -> Mux1/2
  Mux1/1 -> x[k]/1
  Mux2/1 -> x.sat/1
  [x2_xSat] -> Mux2/2
  [x1_xSat] -> Mux2/1
  [x1_kp1] -> x1/2(u[k+1])
  [reset] -> x1/4(reset)
  x1/1(u[k]) -> [x1]
  x1/2(x.sat) -> [x1_xSat]
  [x1_max] -> x1/1(u.max)
  [x1_min] -> x1/3(u.min)
  max(K•C•x)/1 -> Limits Calculation/1(max(K•C•x))
  min(K•C•x)/1 -> Limits Calculation/2(min(K•C•x))
  [x2] -> Unit Delay/1
  Limits Calculation/1(x1.max) -> [x1_max]
  Limits Calculation/2(x2.max) -> [x2_max]
  Limits Calculation/3(x1.min) -> [x1_min]
  Limits Calculation/4(x2.min) -> [x2_min]
  [x2_min] -> x2/3(u.min)
  [x2_max] -> x2/1(u.max)
  x2/2(x.sat) -> [x2_xSat]
  x2/1(u[k]) -> [x2]
  [reset] -> x2/4(reset)
  [x2_kp1] -> x2/2(u[k+1])
  reset/1 -> [reset]
  [x1] -> Limits Calculation/3(x1)
  Unit Delay/1 -> Limits Calculation/4(x2)

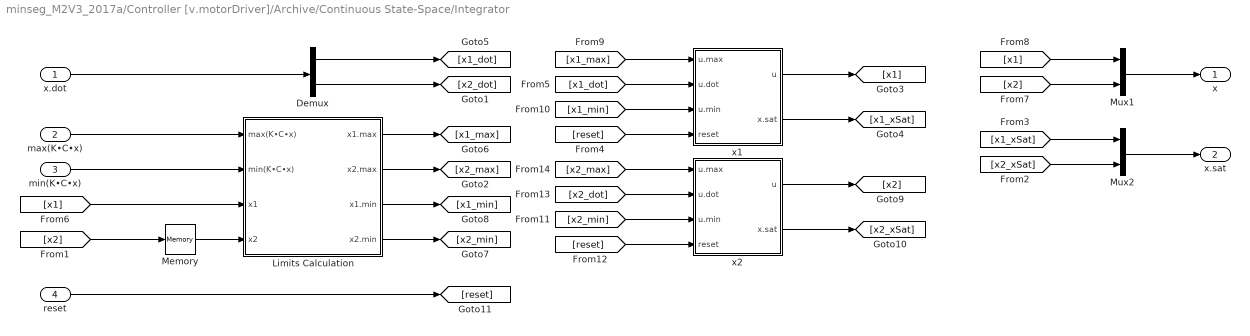
== system minseg_M2V3_2017a/Controller [v.motorDriver]/Archive/Continuous State-Space/Integrator ==
  x.dot : Inport
  max(K•C•x) : Inport  Port=2
  min(K•C•x) : Inport  Port=3
  reset : Inport  Port=4
  Demux : Demux  Outputs=2
  Limits Calculation : Subsystem
  Memory : Memory
  Mux1 : Mux  Inputs=2
  Mux2 : Mux  Inputs=2
  x1 : Subsystem  mask{u_init=state_initialCondition(1,1), k_antiWindup=k_antiWindup(1,1)}
      mask prompts: u_init "Initial Condition"; k_antiWindup "Anti-windup Gain"
  x2 : Subsystem  mask{u_init=state_initialCondition(2,1), k_antiWindup=k_antiWindup(2,1)}
      mask prompts: u_init "Initial Condition"; k_antiWindup "Anti-windup Gain"
  x : Outport
  x.sat : Outport  Port=2
  wires:
  Memory/1 -> Limits Calculation/4(x2)
  [x1] -> Limits Calculation/3(x1)
  reset/1 -> [reset]
  [x2_dot] -> x2/2(u.dot)
  [reset] -> x2/4(reset)
  x2/1(u) -> [x2]
  x2/2(x.sat) -> [x2_xSat]
  [x2_max] -> x2/1(u.max)
  [x2_min] -> x2/3(u.min)
  Limits Calculation/4(x2.min) -> [x2_min]
  Limits Calculation/3(x1.min) -> [x1_min]
  Limits Calculation/2(x2.max) -> [x2_max]
  Limits Calculation/1(x1.max) -> [x1_max]
  [x2] -> Memory/1
  min(K•C•x)/1 -> Limits Calculation/2(min(K•C•x))
  max(K•C•x)/1 -> Limits Calculation/1(max(K•C•x))
  [x1_min] -> x1/3(u.min)
  [x1_max] -> x1/1(u.max)
  x1/2(x.sat) -> [x1_xSat]
  x1/1(u) -> [x1]
  [reset] -> x1/4(reset)
  [x1_dot] -> x1/2(u.dot)
  [x1_xSat] -> Mux2/1
  [x2_xSat] -> Mux2/2
  Mux2/1 -> x.sat/1
  Mux1/1 -> x/1
  [x2] -> Mux1/2
  [x1] -> Mux1/1
  Demux/2 -> [x2_dot]
  Demux/1 -> [x1_dot]
  x.dot/1 -> Demux/1

== system minseg_M2V3_2017a/Controller [v.motorDriver]/Controller and Enable/Controller/Feed-Forward ==
  userIO.read.controller.command : Inport
  Bus Selector1 : BusSelector  OutputSignals=left.motorDriver_v [V],middle.motorDriver_v [V]
  Mux1 : Mux  Inputs=2
  Pass-Through : Subsystem
  output : Outport
  wires:
  userIO.read.controller.command/1 -> Bus Selector1/1
  Mux1/1 -> output/1
  Bus Selector1/1 -> Pass-Through/1(In1)  "<motorDriver_v [V]>"
  Bus Selector1/2 -> Pass-Through/2(In2)  "<motorDriver_v [V]>"
  Pass-Through/1(Out1) -> Mux1/1
  Pass-Through/2(Out2) -> Mux1/2

== system minseg_M2V3_2017a/Controller [v.motorDriver]/Controller and Enable/Controller/PID ==
  userIO.read.controller.command : Inport
  plant.angularVelocity.wheel.body.left : Inport  Port=2
  plant.angularVelocity.wheel.body.middle : Inport  Port=3
  Bus Creator{6,8..10,14..15} (6 alike) : BusCreator  Inputs=1
  Bus Creator7 : BusCreator  Inputs=2
  Bus Selector1 : BusSelector  OutputSignals=left.theta_global_average_dot [rad/s],middle.theta_global_average_dot [rad/s]
  Left-Connected Motor : Subsystem
  Middle-Connected Motor : Subsystem
  Mux1 : Mux  Inputs=2
  output : Outport
  error : Outport  Port=2
  wires:
  userIO.read.controller.command/1 -> Bus Selector1/1
  plant.angularVelocity.wheel.body.left/1 -> Left-Connected Motor/2(measured)
  plant.angularVelocity.wheel.body.middle/1 -> Middle-Connected Motor/2(measured)
  Bus Selector1/1 -> Left-Connected Motor/1(command)  "<theta_global_average_dot [rad/s]>"
  Bus Selector1/2 -> Middle-Connected Motor/1(command)  "<theta_global_average_dot [rad/s]>"
  [e_left] -> Bus Creator14/1  "angularVelocity [rad/s]"
  [e_middle] -> Bus Creator15/1  "angularVelocity [rad/s]"
  Mux1/1 -> output/1
  Bus Creator7/1 -> error/1
  Bus Creator14/1 -> Bus Creator7/1  "left"
  Bus Creator15/1 -> Bus Creator7/2  "middle"
  [v_left] -> Bus Creator8/1  "command [V]"
  Bus Creator8/1 -> Bus Creator6/1  "voltage"
  Bus Creator6/1 -> Mux1/1
  Bus Creator9/1 -> Mux1/2
  Bus Creator10/1 -> Bus Creator9/1  "voltage"
  [v_middle] -> Bus Creator10/1  "command [V]"
  Left-Connected Motor/1(output) -> [v_left]
  Left-Connected Motor/2(error) -> [e_left]
  Middle-Connected Motor/1(output) -> [v_middle]
  Middle-Connected Motor/2(error) -> [e_middle]

== system minseg_M2V3_2017a/Controller [v.motorDriver]/Controller and Enable/Controller/State Feedback Regulation ==
  userIO.read.controller.command : Inport
  plant.state : Inport  Port=2
  Add : Sum  Inputs=-+
  Gain : Gain  Gain=ctrl_motorDriver_v_sfr_K  Multiplication=Matrix(K*u)
      settings: AttributesFormatString=%<Gain>
  Gain1 : Gain  Gain=-1
  bus2mux [Command] : Subsystem
  bus2mux [State] : Subsystem
  mux2bus [error] : Subsystem
  output : Outport
  error : Outport  Port=2
  wires:
  userIO.read.controller.command/1 -> bus2mux [Command]/1(bus)
  bus2mux [Command]/1(mux) -> Add/1  "reference"
  plant.state/1 -> bus2mux [State]/1(bus)
  bus2mux [State]/1(mux) -> Add/2  "state"
  Add/1 -> Gain/1, mux2bus [error]/1(mux)
  Gain/1 -> Gain1/1  "plant"
  mux2bus [error]/1(bus) -> error/1
  Gain1/1 -> output/1
